simulink model "serialgyros"  (R2017a)
settings: Solver=ode45  StartTime=0.0  StopTime=inf  RelTol=1e-3  EnableMultiTasking=on
libraries: vrlib x3, sharedtransform x2, instrumentlib x1
settings Model: Creator=EQUIPO  LastModifiedBy=MarioAndres
settings OptimizationCC: LifeSpan=inf
settings DebuggingCC: SFUnexpectedBacktrackingDiag=warning  SFNoUnconditionalDefaultTransitionDiag=warning  SFExecutionAtInitializationDiag=none
settings GRTTargetCC: TargetLangStandard=C89/C90 (ANSI)  GeneratePreprocessorConditionals=Disable all
settings ConfigComp: CovMetricSettings=dw  CovHtmlReporting=on  CovSaveCumulativeToWorkspaceVar=on  CovSaveSingleToWorkspaceVar=on  CovExternalEMLEnable=off

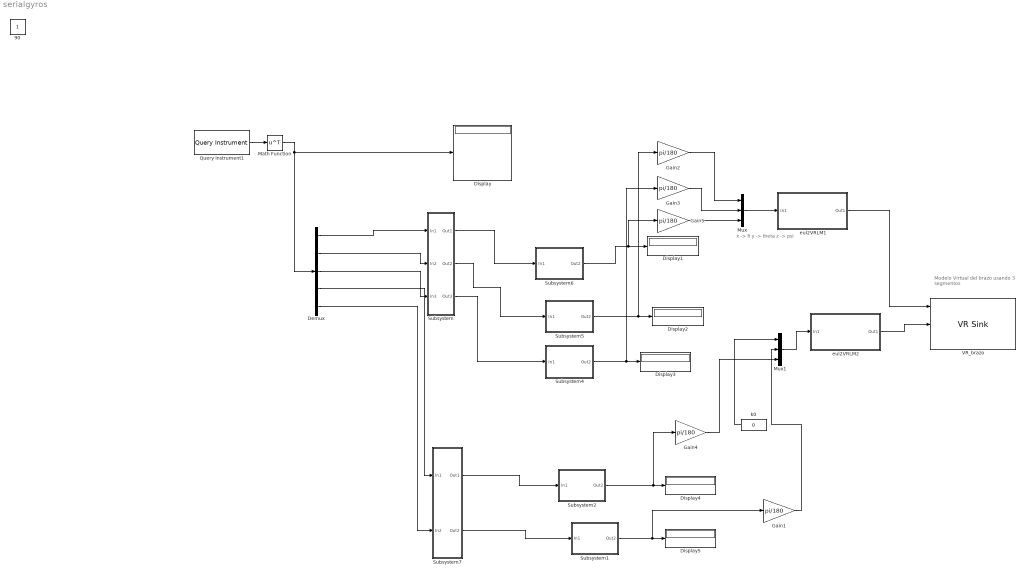
== system serialgyros ==
  note: x -> fi
      | y -> theta
      | z -> psi
  note: Modelo Virtual del brazo
      | usando 3 segmentos
  Demux : Demux  Outputs=5
  Display{,1..5} (6 alike) : Display
  Gain{1..5} (5 alike) : Gain  Gain=pi/180
  Math Function : Math  Operator=transpose  OutputSignalType=real  SaturateOnIntegerOverflow=on
  Mux : Mux  Inputs=3
  Mux1 : Mux  Inputs=3
  Query Instrument1 : instrumentlib/Query Instrument  sampleTime=0.01  isWorkspaceObject=off  timeout=20  inputBufferSize=512  protocol=Serial  serialPort=COM1  baudRate=250000  gpibVendor=Agilent Technologies  boardIndex=0  primaryAddress=1  secondaryAddress=0  visaVendor=Agilent  visaSerialPort=0  chassisIndex=0  logicalAddress=0  tcpRemoteHost='127.0.0.1'  tcpRemotePort=4500  udpRemoteHost='127.0.0.1'  udpRemotePort=9090  visaTCPBoardIndex=0  visaTCPRemoteHost='127.0.0.1'  usbBoardIndex=0  usbManufID=0  usbModelCode=0  usbSerialNumber=0  initAction=None  initCommand='DATA:SOURCE CH1'  initFunction=get  queryCommand='1'  responseFormat=ASCII  asciiFormatting='%d,'  precision=8-bit integer  byteOrder=Little endian  valuesToRead=1  removeBytes=on  afterOutputAction=Repeat query for new data  enableFrames=on  frameSize=5
      settings: SourceProductName=Instrument Control Toolbox  SourceProductBaseCode=IC
  Subsystem : Subsystem
  Subsystem1 : Subsystem
  Subsystem2 : Subsystem
  Subsystem4 : Subsystem
  Subsystem5 : Subsystem
  Subsystem6 : Subsystem
  Subsystem7 : Subsystem
  VR_brazo : vrlib/VR Sink  InstantiateOnLoad=on  SampleTime=0.1  ViewEnable=on  RemoteChange=off  RemoteView=off  FieldsWritten=H.rotation.4.1.1.double#C.rotation.4.1.1.double#M.rotation.4.1.1.double  WorldFileName=Brazo_1.WRL  AutoView=off  VideoDimensions=[]  AllowVariableSize=off  FigureProperties="{'Position', 'Name', 'Viewpoint', 'CameraBound', 'CameraDirection', 'CameraPosition', 'CameraUpVector', 'ZoomFactor', 'Antialiasing', 'Headlight', 'Lighting', 'NavPanel', 'Sound', 'StatusBar', 'Stereo3D', 'Stereo3DCameraOffset', 'Stereo3DHIT', 'ToolBar', 'Textures', 'Transparency', 'Triad', 'Wireframe', 'NavZones', 'NavMode', 'NavSpeed', 'CaptureFileFormat', 'CaptureFileName', 'Record2DCompressMethod', 'Record2DCompressQuality', 'Record2D', 'Record2DFileName', 'Record2DFPS'; [5.0000000000000000e+00   9.2000000000000000e+01   5.7600000000000000e+02   3.5000000000000000e+02], '', '_untitled_1', 'on', [0.0000000000000000e+00   0.0000000000000000e+00  -1.0000000000000000e+00], [0.0000000000000000e+00   0.0000000000000000e+00   0.0000000000000000e+00], [0.0000000000000000e+00   1.0000000000000000e+00   0.0000000000000000e+00], [1.0000000000000000e+00], 'on', 'on', 'on', 'halfbar', 'on', 'on', 'off', [1.0000000149011612e-01], [0.0000000000000000e+00], 'on', 'on', 'on', 'none', 'off', 'off', 'fly', 'normal', 'tif', '%f_anim_%n.tif', 'auto', [7.5000000000000000e+01], 'off', '%f_anim_%n.avi', 'auto'}"
      settings: SourceProductBaseCode=VR
  eul2VRLM1 : Subsystem
  eul2VRLM2 : Subsystem
  k0 : Constant  Value=0
  90 : Constant  IOType=siggen
  wires:
  Query Instrument1/1 -> Math Function/1
  Math Function/1 -> Demux/1, Display/1
  Subsystem2/1(Out2) -> Gain4/1, Display4/1
  Subsystem1/1(Out2) -> Gain1/1, Display5/1
  Demux/1 -> Subsystem/1(In1)
  Demux/2 -> Subsystem/2(In2)
  Demux/3 -> Subsystem/3(In3)
  Subsystem/1(Out1) -> Subsystem6/1(In1)
  Subsystem/2(Out2) -> Subsystem5/1(In1)
  Subsystem/3(Out3) -> Subsystem4/1(In1)
  Demux/4 -> Subsystem7/1(In1)
  Demux/5 -> Subsystem7/2(In2)
  Subsystem7/1(Out1) -> Subsystem2/1(In1)
  Subsystem7/2(Out2) -> Subsystem1/1(In1)
  Mux1/1 -> eul2VRLM2/1(In1)
  Subsystem5/1(Out2) -> Gain2/1, Display2/1
  Subsystem4/1(Out2) -> Gain3/1, Display3/1
  Subsystem6/1(Out2) -> Gain5/1, Display1/1
  eul2VRLM2/1(Out1) -> VR_brazo/2
  eul2VRLM1/1(Out1) -> VR_brazo/1
  Mux/1 -> eul2VRLM1/1(In1)
  Gain1/1 -> Mux1/2
  Gain2/1 -> Mux/1
  Gain3/1 -> Mux/2
  Gain5/1 -> Mux/3
  k0/1 -> Mux1/1
  Gain4/1 -> Mux1/3

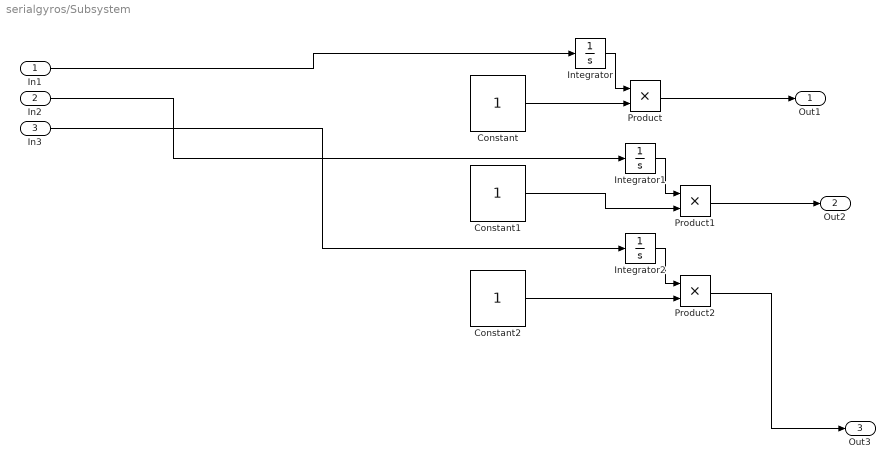
== system serialgyros/Subsystem ==
  In1 : Inport
  In2 : Inport  Port=2
  In3 : Inport  Port=3
  Constant : Constant
  Constant1 : Constant
  Constant2 : Constant
  Integrator : Integrator
  Integrator1 : Integrator
  Integrator2 : Integrator
  Product : Product
  Product1 : Product
  Product2 : Product
  Out1 : Outport
  Out2 : Outport  Port=2
  Out3 : Outport  Port=3
  wires:
  In1/1 -> Integrator/1
  In3/1 -> Integrator2/1
  Constant/1 -> Product/2
  Integrator/1 -> Product/1
  Integrator1/1 -> Product1/1
  Constant1/1 -> Product1/2
  In2/1 -> Integrator1/1
  Constant2/1 -> Product2/2
  Integrator2/1 -> Product2/1
  Product/1 -> Out1/1
  Product1/1 -> Out2/1
  Product2/1 -> Out3/1

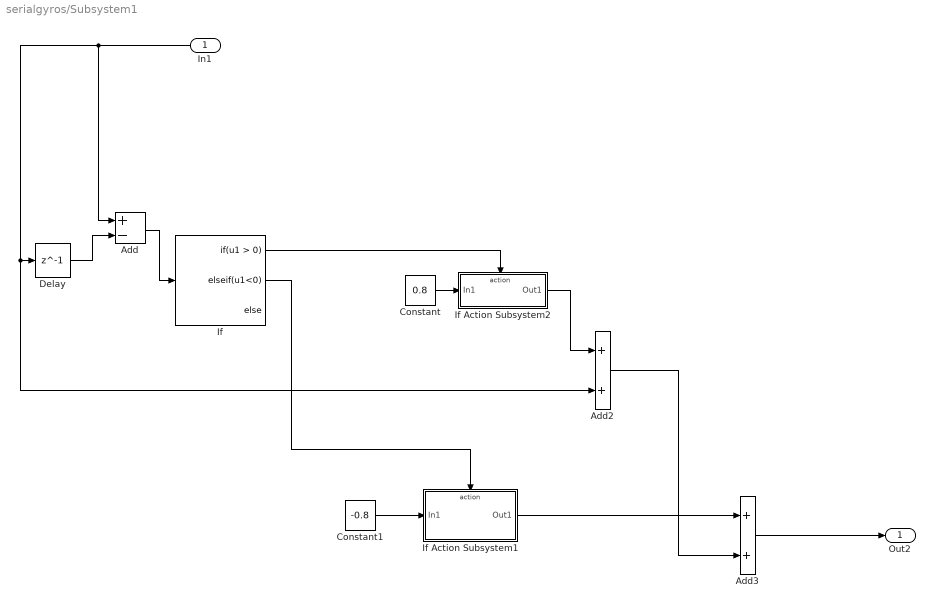
== system serialgyros/Subsystem1 ==
  In1 : Inport
  Add : Sum  Inputs=+-
  Add2 : Sum
  Add3 : Sum
  Constant : Constant  Value=0.8
  Constant1 : Constant  Value=-0.8
  Delay : Delay  DelayLength=1  InitialCondition=0  SampleTime=0.01
  If : If  ElseIfExpressions=u1<0
  If Action Subsystem1 : Subsystem  TreatAsAtomicUnit=on
  If Action Subsystem2 : Subsystem  TreatAsAtomicUnit=on
  Out2 : Outport
  wires:
  Delay/1 -> Add/2
  If/1 -> If Action Subsystem2/Action
  Add/1 -> If/1
  If/2 -> If Action Subsystem1/Action
  If Action Subsystem1/1(Out1) -> Add3/1
  Add2/1 -> Add3/2
  Constant1/1 -> If Action Subsystem1/1(In1)
  Add3/1 -> Out2/1
  Constant/1 -> If Action Subsystem2/1(In1)
  If Action Subsystem2/1(Out1) -> Add2/1
  In1/1 -> Add/1, Add2/2, Delay/1

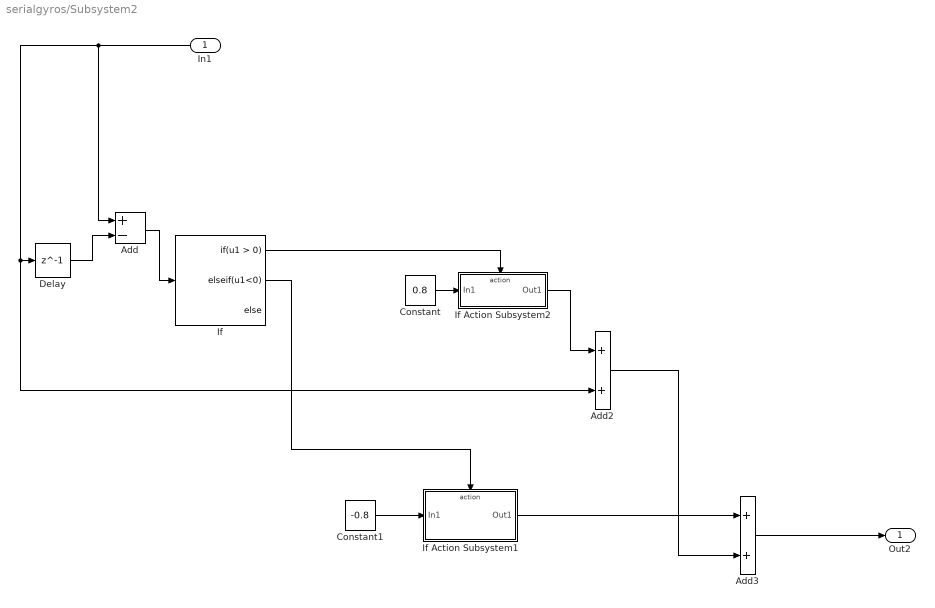
== system serialgyros/Subsystem2 ==
  In1 : Inport
  Add : Sum  Inputs=+-
  Add2 : Sum
  Add3 : Sum
  Constant : Constant  Value=0.8
  Constant1 : Constant  Value=-0.8
  Delay : Delay  DelayLength=1  InitialCondition=0  SampleTime=0.01
  If : If  ElseIfExpressions=u1<0
  If Action Subsystem1 : Subsystem  TreatAsAtomicUnit=on
  If Action Subsystem2 : Subsystem  TreatAsAtomicUnit=on
  Out2 : Outport
  wires:
  In1/1 -> Delay/1, Add2/2, Add/1
  If Action Subsystem2/1(Out1) -> Add2/1
  Constant/1 -> If Action Subsystem2/1(In1)
  Add3/1 -> Out2/1
  Constant1/1 -> If Action Subsystem1/1(In1)
  Add2/1 -> Add3/2
  If Action Subsystem1/1(Out1) -> Add3/1
  If/2 -> If Action Subsystem1/Action
  Add/1 -> If/1
  If/1 -> If Action Subsystem2/Action
  Delay/1 -> Add/2

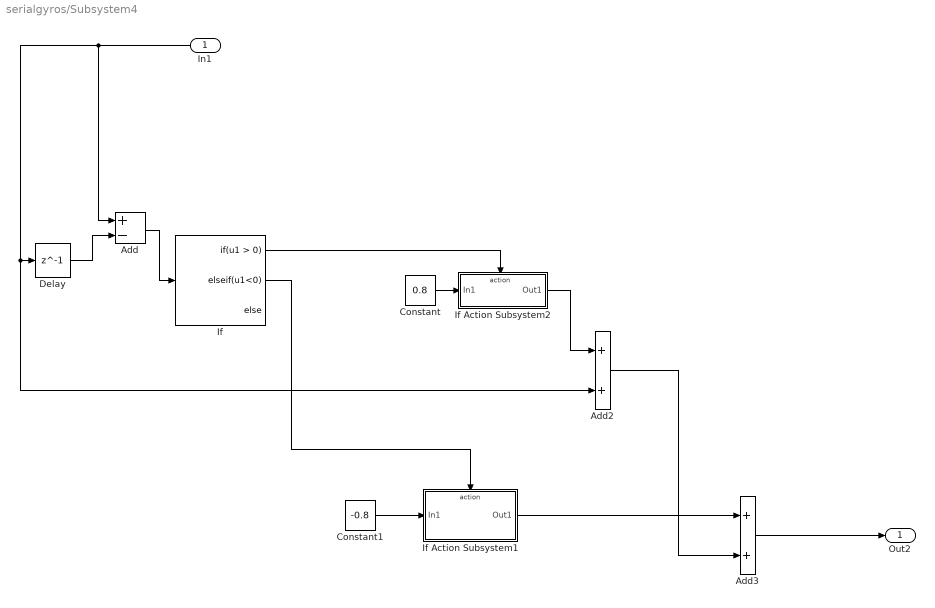
== system serialgyros/Subsystem4 ==
  In1 : Inport
  Add : Sum  Inputs=+-
  Add2 : Sum
  Add3 : Sum
  Constant : Constant  Value=0.8
  Constant1 : Constant  Value=-0.8
  Delay : Delay  DelayLength=1  InitialCondition=0  SampleTime=0.01
  If : If  ElseIfExpressions=u1<0
  If Action Subsystem1 : Subsystem  TreatAsAtomicUnit=on
  If Action Subsystem2 : Subsystem  TreatAsAtomicUnit=on
  Out2 : Outport
  wires:
  Delay/1 -> Add/2
  If/1 -> If Action Subsystem2/Action
  Add/1 -> If/1
  If/2 -> If Action Subsystem1/Action
  If Action Subsystem1/1(Out1) -> Add3/1
  Add2/1 -> Add3/2
  Constant1/1 -> If Action Subsystem1/1(In1)
  Add3/1 -> Out2/1
  Constant/1 -> If Action Subsystem2/1(In1)
  If Action Subsystem2/1(Out1) -> Add2/1
  In1/1 -> Add/1, Add2/2, Delay/1

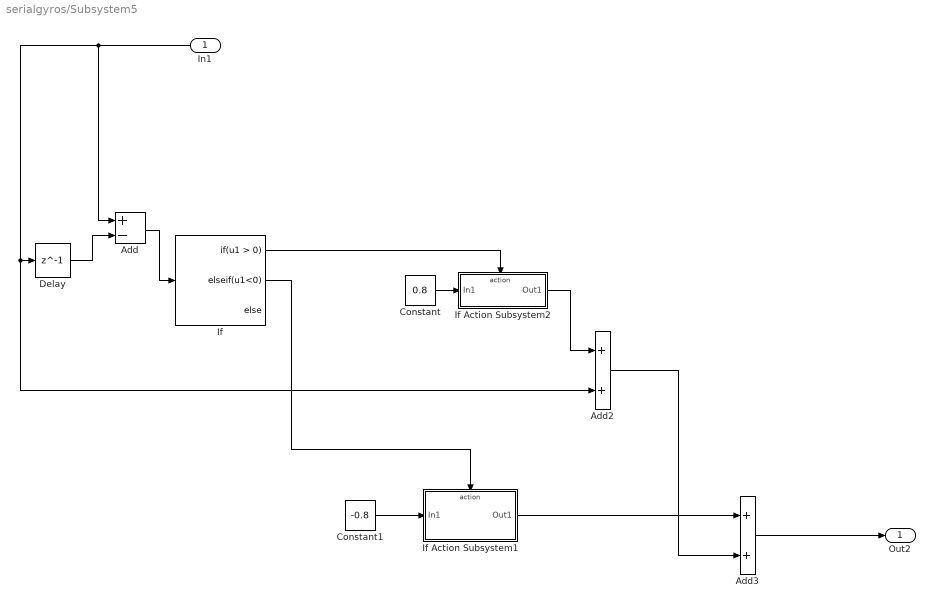
== system serialgyros/Subsystem5 ==
  In1 : Inport
  Add : Sum  Inputs=+-
  Add2 : Sum
  Add3 : Sum
  Constant : Constant  Value=0.8
  Constant1 : Constant  Value=-0.8
  Delay : Delay  DelayLength=1  InitialCondition=0  SampleTime=0.01
  If : If  ElseIfExpressions=u1<0
  If Action Subsystem1 : Subsystem  TreatAsAtomicUnit=on
  If Action Subsystem2 : Subsystem  TreatAsAtomicUnit=on
  Out2 : Outport
  wires:
  In1/1 -> Delay/1, Add2/2, Add/1
  If Action Subsystem2/1(Out1) -> Add2/1
  Constant/1 -> If Action Subsystem2/1(In1)
  Add3/1 -> Out2/1
  Constant1/1 -> If Action Subsystem1/1(In1)
  Add2/1 -> Add3/2
  If Action Subsystem1/1(Out1) -> Add3/1
  If/2 -> If Action Subsystem1/Action
  Add/1 -> If/1
  If/1 -> If Action Subsystem2/Action
  Delay/1 -> Add/2

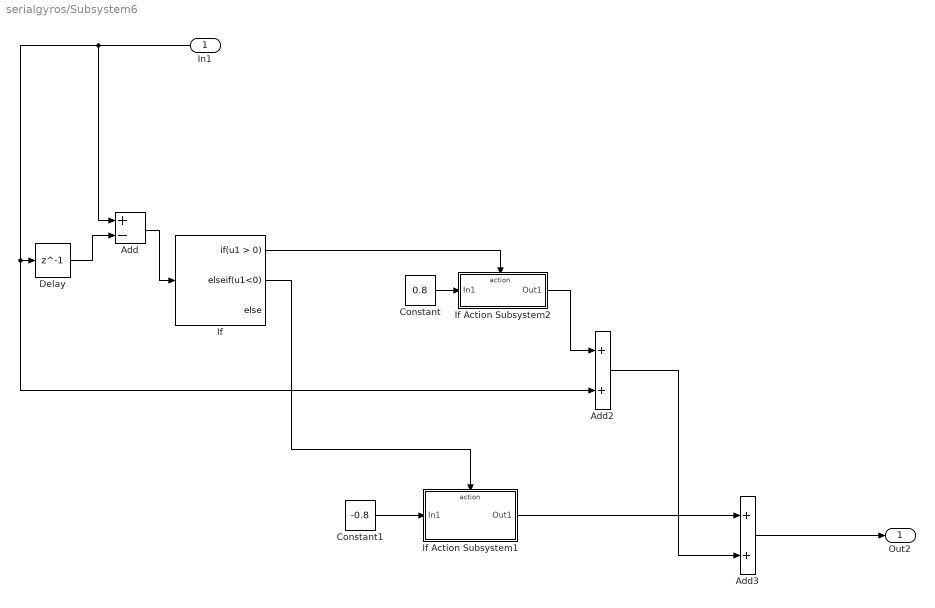
== system serialgyros/Subsystem6 ==
  In1 : Inport
  Add : Sum  Inputs=+-
  Add2 : Sum
  Add3 : Sum
  Constant : Constant  Value=0.8
  Constant1 : Constant  Value=-0.8
  Delay : Delay  DelayLength=1  InitialCondition=0  SampleTime=0.01
  If : If  ElseIfExpressions=u1<0
  If Action Subsystem1 : Subsystem  TreatAsAtomicUnit=on
  If Action Subsystem2 : Subsystem  TreatAsAtomicUnit=on
  Out2 : Outport
  wires:
  Delay/1 -> Add/2
  If/1 -> If Action Subsystem2/Action
  Add/1 -> If/1
  If/2 -> If Action Subsystem1/Action
  If Action Subsystem1/1(Out1) -> Add3/1
  Add2/1 -> Add3/2
  Constant1/1 -> If Action Subsystem1/1(In1)
  Add3/1 -> Out2/1
  Constant/1 -> If Action Subsystem2/1(In1)
  If Action Subsystem2/1(Out1) -> Add2/1
  In1/1 -> Add/1, Add2/2, Delay/1

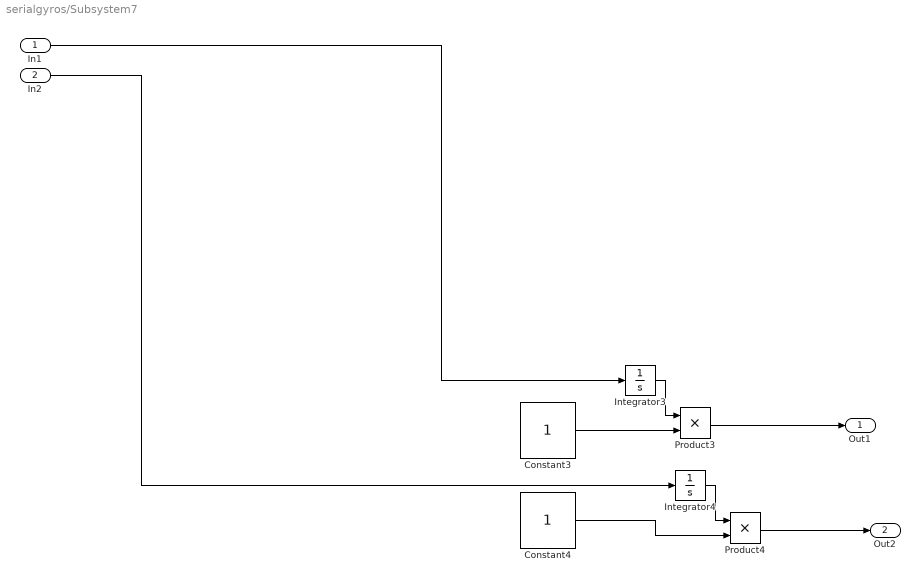
== system serialgyros/Subsystem7 ==
  In1 : Inport
  In2 : Inport  Port=2
  Constant3 : Constant
  Constant4 : Constant
  Integrator3 : Integrator
  Integrator4 : Integrator
  Product3 : Product
  Product4 : Product
  Out1 : Outport
  Out2 : Outport  Port=2
  wires:
  Product4/1 -> Out2/1
  Product3/1 -> Out1/1
  In2/1 -> Integrator4/1
  Constant4/1 -> Product4/2
  Integrator4/1 -> Product4/1
  Integrator3/1 -> Product3/1
  Constant3/1 -> Product3/2
  In1/1 -> Integrator3/1

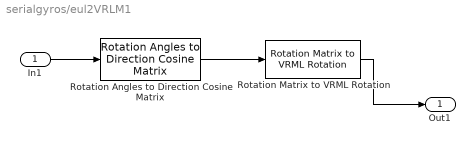
== system serialgyros/eul2VRLM1 ==
  In1 : Inport
  Rotation Angles to Direction Cosine Matrix : sharedtransform/Rotation Angles to Direction Cosine Matrix  rotationOrder=ZYX
  Rotation Matrix to VRML Rotation : vrlib/Utilities/Rotation Matrix to VRML Rotation  maxzero=1e-12
      settings: SourceProductName=Simulink 3D Animation  SourceProductBaseCode=VR
  Out1 : Outport
  wires:
  Rotation Matrix to VRML Rotation/1 -> Out1/1
  In1/1 -> Rotation Angles to Direction Cosine Matrix/1
  Rotation Angles to Direction Cosine Matrix/1 -> Rotation Matrix to VRML Rotation/1

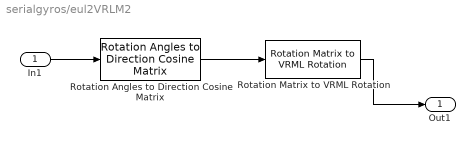
== system serialgyros/eul2VRLM2 ==
  In1 : Inport
  Rotation Angles to Direction Cosine Matrix : sharedtransform/Rotation Angles to Direction Cosine Matrix  rotationOrder=ZYX
  Rotation Matrix to VRML Rotation : vrlib/Utilities/Rotation Matrix to VRML Rotation  maxzero=1e-12
      settings: SourceProductName=Simulink 3D Animation  SourceProductBaseCode=VR
  Out1 : Outport
  wires:
  Rotation Angles to Direction Cosine Matrix/1 -> Rotation Matrix to VRML Rotation/1
  In1/1 -> Rotation Angles to Direction Cosine Matrix/1
  Rotation Matrix to VRML Rotation/1 -> Out1/1

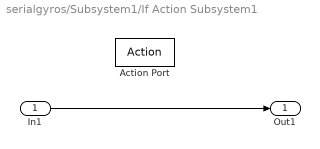
== system serialgyros/Subsystem1/If Action Subsystem1 ==
  In1 : Inport
  Action Port : ActionPort  ActionType=elseif
  Out1 : Outport
  wires:
  In1/1 -> Out1/1

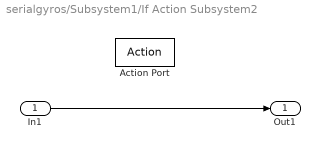
== system serialgyros/Subsystem1/If Action Subsystem2 ==
  In1 : Inport
  Action Port : ActionPort  ActionType=then
  Out1 : Outport
  wires:
  In1/1 -> Out1/1

== system serialgyros/Subsystem2/If Action Subsystem1 ==
  In1 : Inport
  Action Port : ActionPort  ActionType=elseif
  Out1 : Outport
  wires:
  In1/1 -> Out1/1

== system serialgyros/Subsystem2/If Action Subsystem2 ==
  In1 : Inport
  Action Port : ActionPort  ActionType=then
  Out1 : Outport
  wires:
  In1/1 -> Out1/1

== system serialgyros/Subsystem4/If Action Subsystem1 ==
  In1 : Inport
  Action Port : ActionPort  ActionType=elseif
  Out1 : Outport
  wires:
  In1/1 -> Out1/1

== system serialgyros/Subsystem4/If Action Subsystem2 ==
  In1 : Inport
  Action Port : ActionPort  ActionType=then
  Out1 : Outport
  wires:
  In1/1 -> Out1/1

== system serialgyros/Subsystem5/If Action Subsystem1 ==
  In1 : Inport
  Action Port : ActionPort  ActionType=elseif
  Out1 : Outport
  wires:
  In1/1 -> Out1/1

== system serialgyros/Subsystem5/If Action Subsystem2 ==
  In1 : Inport
  Action Port : ActionPort  ActionType=then
  Out1 : Outport
  wires:
  In1/1 -> Out1/1

== system serialgyros/Subsystem6/If Action Subsystem1 ==
  In1 : Inport
  Action Port : ActionPort  ActionType=elseif
  Out1 : Outport
  wires:
  In1/1 -> Out1/1

== system serialgyros/Subsystem6/If Action Subsystem2 ==
  In1 : Inport
  Action Port : ActionPort  ActionType=then
  Out1 : Outport
  wires:
  In1/1 -> Out1/1
